simulink model "actuator_simplified_to_first_order"  (R2025b)
settings: Solver=VariableStepAuto  StartTime=0.0  StopTime=10.0  MaxStep=1e-3  RelTol=1e-3
model workspace (MAT data in the model file):
  damping = Simulink.Parameter
  damping.Value = 0.795
  damping.Complexity = 'real'
  damping.Dimensions = [1 1]
  damping.DataType = 'auto'
  omega_nat = Simulink.Parameter
  omega_nat.Value = 7.2225
  omega_nat.Complexity = 'real'
  omega_nat.Dimensions = [1 1]
  omega_nat.DataType = 'auto'
libraries: eeGeneralControl x1
settings Model: Creator=karadeli  LastModifiedBy=karadeli

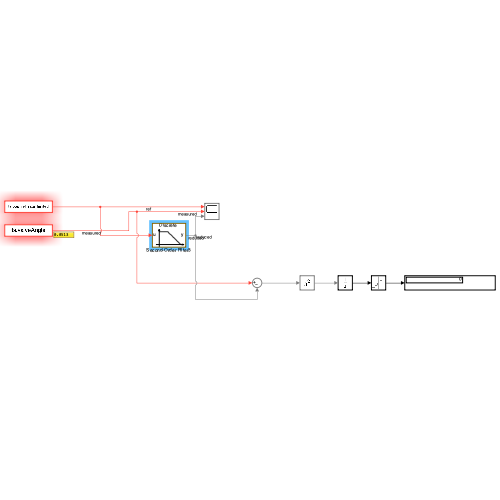
[thumbnail: Simulink's stored preview of the top-level diagram]
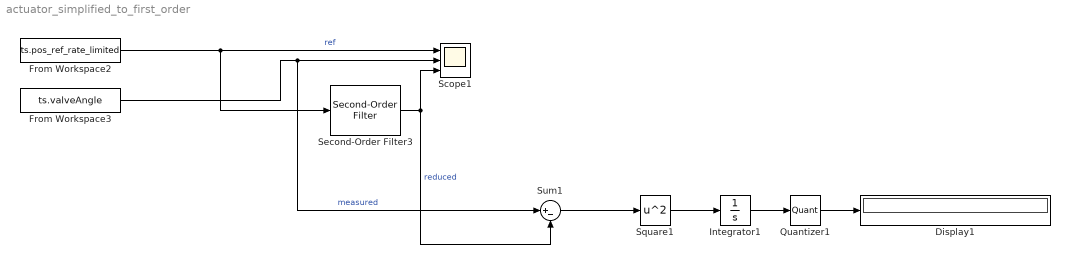
== system actuator_simplified_to_first_order ==
  Display1 : Display
      settings: Decimation=3
  From Workspace2 : FromWorkspace  VariableName=ts.pos_ref_rate_limited  SampleTime=1e-3  Interpolate=off  OutputAfterFinalValue=Setting to zero
  From Workspace3 : FromWorkspace  VariableName=ts.valveAngle  SampleTime=1e-3  Interpolate=off  OutputAfterFinalValue=Setting to zero
  Integrator1 : Integrator
  Quantizer1 : Quantizer  QuantizationInterval=0.0001
  Scope1 : Scope  NumInputPorts=3
      settings: ActiveDisplayYMinimum=-18.977052110650419  ActiveDisplayYMaximum=169.20221899845686
  Second-Order Filter3 : eeGeneralControl/Second-Order Filter  FilterType=Low-pass  fn=21.64  Zeta=0.86  Ts=-1  A0=0  Ph0=0  f0=0  b0=0
      settings: LibrarySourceBlock=ee_sl_lib/General Control/Second-Order Filter
  Square1 : Math  Operator=square
  Sum1 : Sum  Inputs=|+-
  wires:
  From Workspace2/1 -> Second-Order Filter3/1, Scope1/1  "ref"
  From Workspace3/1 -> Scope1/2, Sum1/1  "measured"
  Square1/1 -> Integrator1/1
  Sum1/1 -> Square1/1
  Second-Order Filter3/1 -> Sum1/2, Scope1/3  "reduced"
  Quantizer1/1 -> Display1/1
  Integrator1/1 -> Quantizer1/1
